simulink model "LKS_tcp11"  (R2024b)
settings: Solver=VariableStepAuto  StartTime=0.0  StopTime=100  RelTol=1e-3
libraries: simulink x3, simulink_extras x3, instrumentlib x1
settings Model: Creator=28509  LastModifiedBy=zc
settings DataIOCC: SaveFormat=Array  ReturnWorkspaceOutputs=off

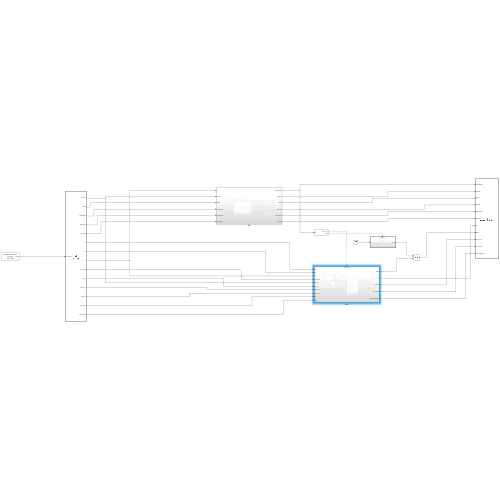
[thumbnail: Simulink's stored preview of the top-level diagram]
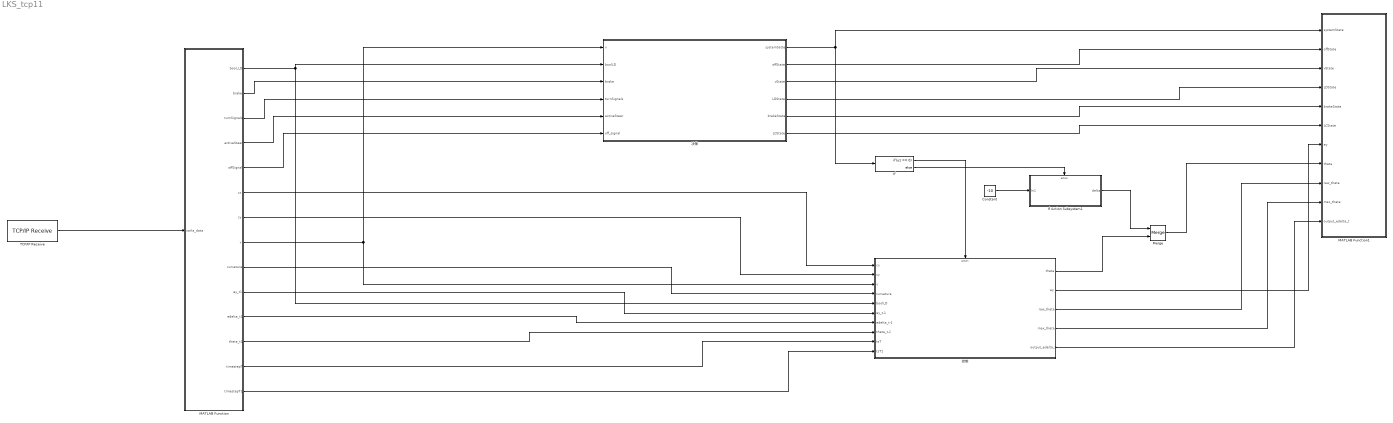
== system LKS_tcp11 ==
  Constant : Constant  Value=-10
  If : If  IfExpression=u1 == 0
  If Action Subsystem1 : Subsystem  TreatAsAtomicUnit=on
  MATLAB Function : MATLAB Function  TreatAsAtomicUnit=on
  MATLAB Function1 : MATLAB Function  TreatAsAtomicUnit=on
  Merge : Merge
  TCP/IP Receive : instrumentlib/TCP//IP Receive  Host=127.0.0.1  Port=25026  DataSize=[ 1, 191]  DataType=double  ASCIIFormatting=%f  Terminator=LF  CustomTerminator=10  ByteOrder=little-endian  EnableBlockingMode=on  Timeout=5  SampleTime=0.01  SimulateUsing=Interpreted execution
  决策 : Subsystem
  控制 : Subsystem  TreatAsAtomicUnit=on
  wires:
  控制/1(theta) -> Merge/2
  MATLAB Function/2(brake) -> 决策/3(brake)
  MATLAB Function/3(turnSignals) -> 决策/4(turnSignals)
  MATLAB Function/4(activeSteer) -> 决策/5(activeSteer)
  决策/1(systemSatte) -> If/1, MATLAB Function1/1(systemState)
  If/1 -> 控制/Action
  MATLAB Function/7(cy) -> 控制/2(cy)
  If/2 -> If Action Subsystem1/Action
  Constant/1 -> If Action Subsystem1/1(In1)
  If Action Subsystem1/1(delta) -> Merge/1
  Merge/1 -> MATLAB Function1/8(theta)
  MATLAB Function/5(offSignal) -> 决策/6(off_signal)
  TCP/IP Receive/1 -> MATLAB Function/1(carla_data)
  MATLAB Function/8(v) -> 决策/1(v), 控制/3(v)
  决策/2(offState) -> MATLAB Function1/2(offState)
  决策/3(vState) -> MATLAB Function1/3(vState)
  决策/4(LDState) -> MATLAB Function1/4(LDState)
  决策/5(brakeState) -> MATLAB Function1/5(brakeState)
  决策/6(LCState) -> MATLAB Function1/6(LCState)
  控制/2(ey) -> MATLAB Function1/7(ey)
  控制/3(raw_theta) -> MATLAB Function1/9(raw_theta)
  控制/4(max_theta) -> MATLAB Function1/10(max_theta)
  MATLAB Function/6(cx) -> 控制/1(cx)
  MATLAB Function/9(curvature) -> 控制/4(curvature)
  MATLAB Function/1(bool_LD) -> 决策/2(boolLD), 控制/5(boolLD)
  控制/5(output_edelta_t) -> MATLAB Function1/11(output_edelta_t)
  MATLAB Function/10(ey_t1) -> 控制/6(ey_t-1)
  MATLAB Function/11(edelta_t1) -> 控制/7(edelta_t-1)
  MATLAB Function/12(theta_t1) -> 控制/8(theta_t-1)
  MATLAB Function/13(timestepT) -> 控制/9(tsT)
  MATLAB Function/14(timestepT1) -> 控制/10(tsT1)

== system LKS_tcp11/If Action Subsystem1 ==
  In1 : Inport
  Action Port : ActionPort  ActionPortLabel=else
  delta : Outport
  wires:
  In1/1 -> delta/1

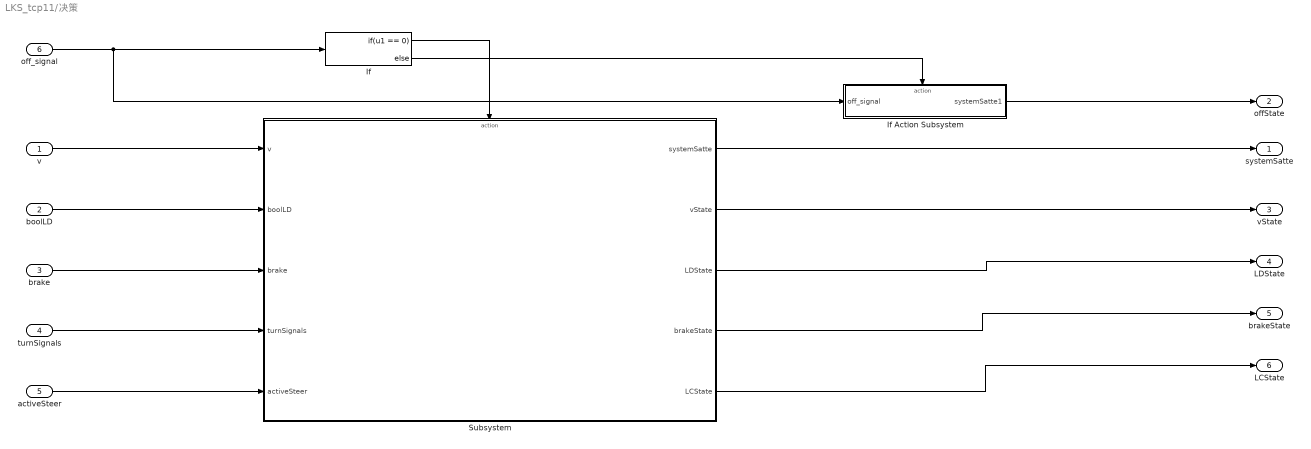
== system LKS_tcp11/决策 ==
  v : Inport
  boolLD : Inport  Port=2
  brake : Inport  Port=3  OutDataTypeStr=double
  turnSignals : Inport  Port=4
  activeSteer : Inport  Port=5
  off_signal : Inport  Port=6
  If : If  IfExpression=u1 == 0
  If Action Subsystem : Subsystem  TreatAsAtomicUnit=on
  Subsystem : Subsystem
  systemSatte : Outport
  offState : Outport  Port=2
  vState : Outport  Port=3
  LDState : Outport  Port=4
  brakeState : Outport  Port=5
  LCState : Outport  Port=6
  wires:
  v/1 -> Subsystem/1(v)
  boolLD/1 -> Subsystem/2(boolLD)
  brake/1 -> Subsystem/3(brake)
  turnSignals/1 -> Subsystem/4(turnSignals)
  activeSteer/1 -> Subsystem/5(activeSteer)
  Subsystem/1(systemSatte) -> systemSatte/1
  If/1 -> Subsystem/Action
  If/2 -> If Action Subsystem/Action
  If Action Subsystem/1(systemSatte1) -> offState/1
  off_signal/1 -> If Action Subsystem/1(off_signal), If/1
  Subsystem/5(LCState) -> LCState/1
  Subsystem/4(brakeState) -> brakeState/1
  Subsystem/2(vState) -> vState/1
  Subsystem/3(LDState) -> LDState/1

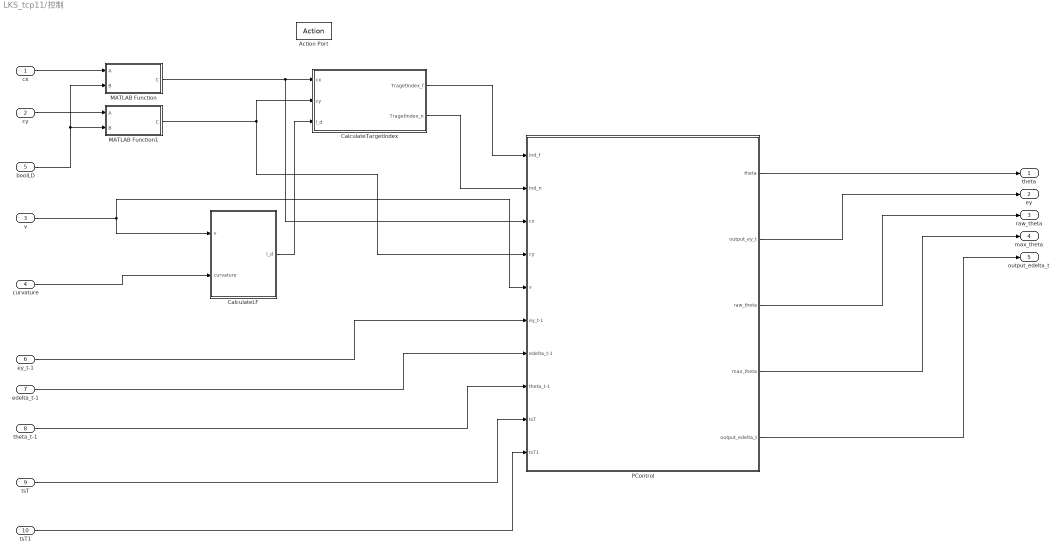
== system LKS_tcp11/控制 ==
  cx : Inport
  cy : Inport  Port=2
  v : Inport  Port=3
  curvature : Inport  Port=4
  boolLD : Inport  Port=5
  ey_t-1 : Inport  Port=6
  edelta_t-1 : Inport  Port=7
  theta_t-1 : Inport  Port=8
  tsT : Inport  Port=9
  tsT1 : Inport  Port=10
  Action Port : ActionPort  ActionPortLabel=if(u1 == 0)
  CalculateLF : Subsystem
  CalculateTargetIndex : Subsystem
  MATLAB Function : MATLAB Function  TreatAsAtomicUnit=on
  MATLAB Function1 : MATLAB Function  TreatAsAtomicUnit=on
  PControl : Subsystem
  theta : Outport  VectorParamsAs1DForOutWhenUnconnected=off
  ey : Outport  Port=2  VectorParamsAs1DForOutWhenUnconnected=off
  raw_theta : Outport  Port=3  VectorParamsAs1DForOutWhenUnconnected=off
  max_theta : Outport  Port=4  VectorParamsAs1DForOutWhenUnconnected=off
  output_edelta_t : Outport  Port=5  VectorParamsAs1DForOutWhenUnconnected=off
  wires:
  PControl/1(theta) -> theta/1
  CalculateLF/1(l_d) -> CalculateTargetIndex/3(l_d)
  CalculateTargetIndex/2(TragetIndex_n) -> PControl/2(ind_n)
  v/1 -> PControl/5(v), CalculateLF/1(v)
  PControl/2(output_ey_t) -> ey/1
  PControl/3(raw_theta) -> raw_theta/1
  PControl/4(max_theta) -> max_theta/1
  curvature/1 -> CalculateLF/2(curvature)
  cx/1 -> MATLAB Function/1(A)
  MATLAB Function/1(C) -> PControl/3(cx), CalculateTargetIndex/1(cx)
  cy/1 -> MATLAB Function1/1(A)
  MATLAB Function1/1(C) -> PControl/4(cy), CalculateTargetIndex/2(cy)
  boolLD/1 -> MATLAB Function/2(B), MATLAB Function1/2(B)
  CalculateTargetIndex/1(TragetIndex_f) -> PControl/1(ind_f)
  ey_t-1/1 -> PControl/6(ey_t-1)
  edelta_t-1/1 -> PControl/7(edelta_t-1)
  theta_t-1/1 -> PControl/8(theta_t-1)
  PControl/5(output_edelta_t) -> output_edelta_t/1
  tsT/1 -> PControl/9(tsT)
  tsT1/1 -> PControl/10(tsT1)

== system LKS_tcp11/决策/If Action Subsystem ==
  off_signal : Inport
  Action Port : ActionPort  ActionPortLabel=else
  systemSatte1 : Outport
  wires:
  off_signal/1 -> systemSatte1/1

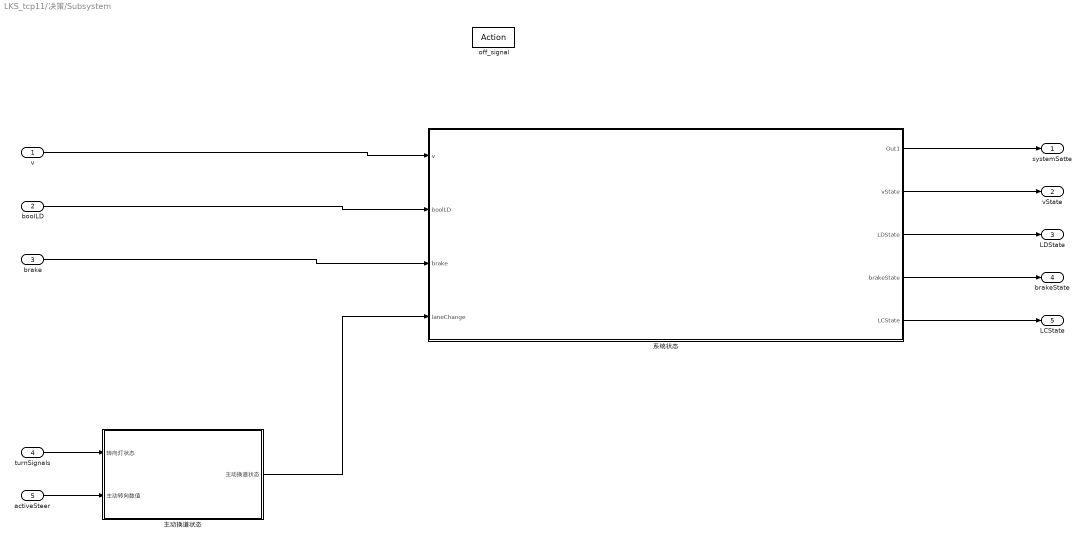
== system LKS_tcp11/决策/Subsystem ==
  v : Inport
  boolLD : Inport  Port=2
  brake : Inport  Port=3  OutDataTypeStr=double
  turnSignals : Inport  Port=4
  activeSteer : Inport  Port=5
  off_signal : ActionPort  ActionPortLabel=if(u1 == 0)
  主动换道状态 : Subsystem
  系统状态 : Subsystem
  systemSatte : Outport
  vState : Outport  Port=2
  LDState : Outport  Port=3
  brakeState : Outport  Port=4
  LCState : Outport  Port=5
  wires:
  v/1 -> 系统状态/1(v)
  主动换道状态/1(主动换道状态) -> 系统状态/4(laneChange)
  turnSignals/1 -> 主动换道状态/1(转向灯状态)
  activeSteer/1 -> 主动换道状态/2(主动转向数值)
  boolLD/1 -> 系统状态/2(boolLD)
  brake/1 -> 系统状态/3(brake)
  系统状态/1(Out1) -> systemSatte/1
  系统状态/2(vState) -> vState/1
  系统状态/3(LDState) -> LDState/1
  系统状态/4(brakeState) -> brakeState/1
  系统状态/5(LCState) -> LCState/1

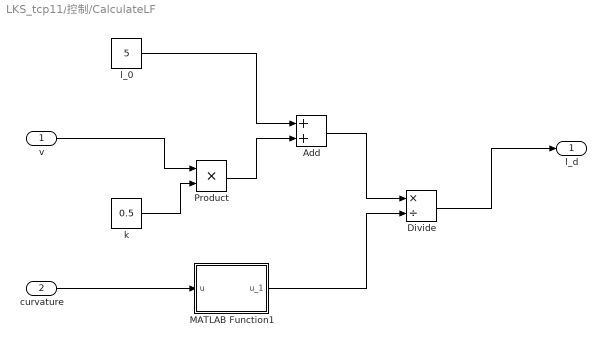
== system LKS_tcp11/控制/CalculateLF ==
  v : Inport
  curvature : Inport  Port=2
  Add : Sum
  Divide : Product  Inputs=*/
  MATLAB Function1 : MATLAB Function  TreatAsAtomicUnit=on
  Product : Product
  k : Constant  Value=0.5
  l_0 : Constant  Value=5
  l_d : Outport
  wires:
  v/1 -> Product/1
  k/1 -> Product/2
  l_0/1 -> Add/1
  Product/1 -> Add/2
  Divide/1 -> l_d/1
  curvature/1 -> MATLAB Function1/1(u)
  Add/1 -> Divide/1
  MATLAB Function1/1(u_1) -> Divide/2

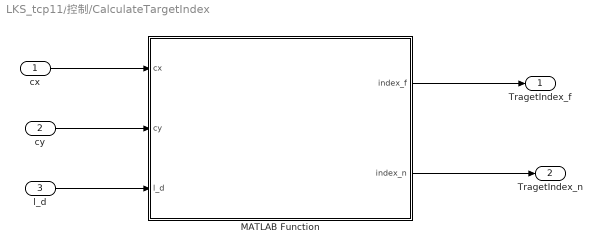
== system LKS_tcp11/控制/CalculateTargetIndex ==
  cx : Inport
  cy : Inport  Port=2
  l_d : Inport  Port=3
  MATLAB Function : MATLAB Function  TreatAsAtomicUnit=on
  TragetIndex_f : Outport
  TragetIndex_n : Outport  Port=2
  wires:
  cx/1 -> MATLAB Function/1(cx)
  cy/1 -> MATLAB Function/2(cy)
  l_d/1 -> MATLAB Function/3(l_d)
  MATLAB Function/2(index_n) -> TragetIndex_n/1
  MATLAB Function/1(index_f) -> TragetIndex_f/1

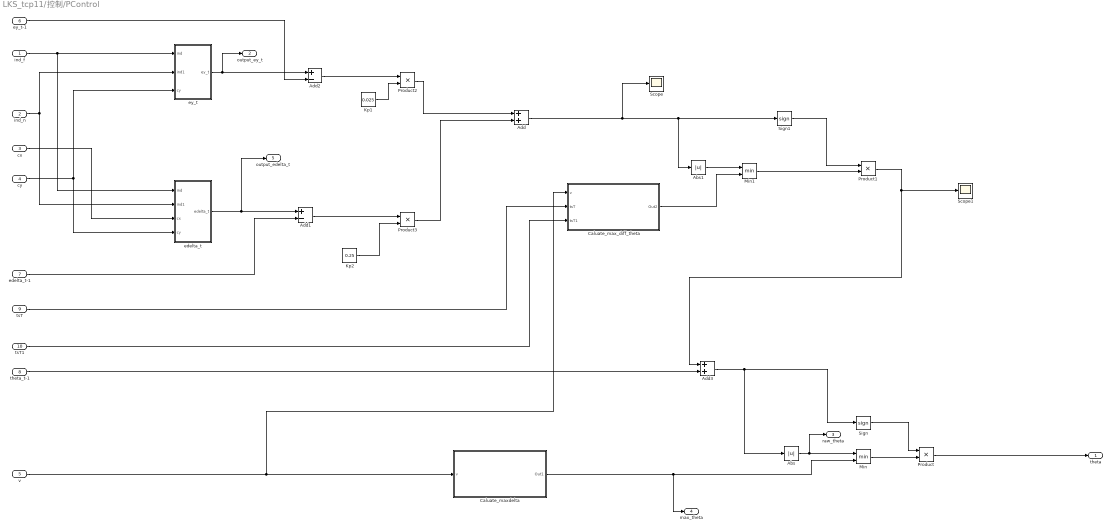
== system LKS_tcp11/控制/PControl ==
  ind_f : Inport
  ind_n : Inport  Port=2
  cx : Inport  Port=3
  cy : Inport  Port=4
  v : Inport  Port=5
  ey_t-1 : Inport  Port=6
  edelta_t-1 : Inport  Port=7
  theta_t-1 : Inport  Port=8
  tsT : Inport  Port=9
  tsT1 : Inport  Port=10
  Abs : Abs  SaturateOnIntegerOverflow=off
  Abs1 : Abs  SaturateOnIntegerOverflow=off
  Add : Sum
  Add1 : Sum  Inputs=+-
  Add2 : Sum  Inputs=+-
  Add3 : Sum
  Caluate_max_diff_theta : Subsystem
  Caluate_maxdelta : Subsystem
  Kp1 : Constant  Value=0.025
  Kp2 : Constant  Value=0.25
  Min : MinMax  Inputs=2
  Min1 : MinMax  Inputs=2
  Product{,1..3} (4 alike) : Product
  Scope : Scope
  Scope1 : Scope
  Sign : Signum
  Sign1 : Signum
  edelta_t : Subsystem
  ey_t : Subsystem
  theta : Outport  VectorParamsAs1DForOutWhenUnconnected=off
  output_ey_t : Outport  Port=2  VectorParamsAs1DForOutWhenUnconnected=off
  raw_theta : Outport  Port=3  VectorParamsAs1DForOutWhenUnconnected=off
  max_theta : Outport  Port=4  VectorParamsAs1DForOutWhenUnconnected=off
  output_edelta_t : Outport  Port=5  VectorParamsAs1DForOutWhenUnconnected=off
  wires:
  Sign/1 -> Product/1
  Min/1 -> Product/2
  Abs/1 -> raw_theta/1, Min/1
  Kp1/1 -> Product2/2
  Product2/1 -> Add/1
  Product3/1 -> Add/2
  Caluate_maxdelta/1(Out1) -> Min/2, max_theta/1
  cy/1 -> edelta_t/4(cy), ey_t/3(cy)
  ind_f/1 -> edelta_t/1(ind), ey_t/1(ind)
  ind_n/1 -> edelta_t/2(ind1), ey_t/2(ind1)
  Kp2/1 -> Product3/2
  cx/1 -> edelta_t/3(cx)
  edelta_t/1(edelta_t) -> output_edelta_t/1, Add1/1
  ey_t/1(ey_t) -> Add2/1, output_ey_t/1
  ey_t-1/1 -> Add2/2
  edelta_t-1/1 -> Add1/2
  Add2/1 -> Product2/1
  Add1/1 -> Product3/1
  Add3/1 -> Abs/1, Sign/1
  Product/1 -> theta/1
  theta_t-1/1 -> Add3/2
  Sign1/1 -> Product1/1
  Min1/1 -> Product1/2
  Abs1/1 -> Min1/1
  Caluate_max_diff_theta/1(Out2) -> Min1/2
  v/1 -> Caluate_maxdelta/1(v), Caluate_max_diff_theta/1(v)
  tsT/1 -> Caluate_max_diff_theta/2(tsT)
  tsT1/1 -> Caluate_max_diff_theta/3(tsT1)
  Add/1 -> Scope/1, Sign1/1, Abs1/1
  Product1/1 -> Scope1/1, Add3/1

== system LKS_tcp11/决策/Subsystem/主动换道状态 ==
  转向灯状态 : Inport
  主动转向数值 : Inport  Port=2
  Abs : Abs  SaturateOnIntegerOverflow=off
  Add : Sum
  Compare To Constant : simulink/Logic and Bit Operations/Compare To Constant  relop=>=  const=0.05  OutDataTypeStr=boolean
  主动换道状态 : Outport
  wires:
  Compare To Constant/1 -> Add/2
  Add/1 -> 主动换道状态/1
  转向灯状态/1 -> Add/1
  主动转向数值/1 -> Abs/1
  Abs/1 -> Compare To Constant/1

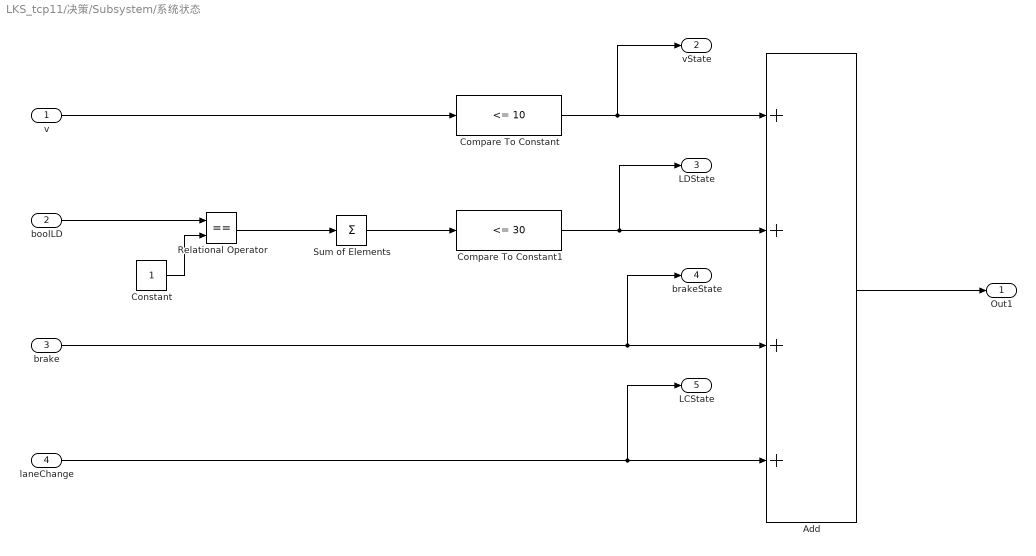
== system LKS_tcp11/决策/Subsystem/系统状态 ==
  v : Inport
  boolLD : Inport  Port=2
  brake : Inport  Port=3
  laneChange : Inport  Port=4
  Add : Sum  Inputs=++++
  Compare To Constant : simulink/Logic and Bit Operations/Compare To Constant  relop=<=  const=10  OutDataTypeStr=boolean
  Compare To Constant1 : simulink/Logic and Bit Operations/Compare To Constant  relop=<=  const=30  OutDataTypeStr=boolean
  Constant : Constant
  Relational Operator : RelationalOperator  Operator===  OutDataTypeStr=boolean  RndMeth=Simplest  InputSameDT=off
  Sum of Elements : Sum  Inputs=+
  Out1 : Outport
  vState : Outport  Port=2
  LDState : Outport  Port=3
  brakeState : Outport  Port=4
  LCState : Outport  Port=5
  wires:
  boolLD/1 -> Relational Operator/1
  Constant/1 -> Relational Operator/2
  Relational Operator/1 -> Sum of Elements/1
  Add/1 -> Out1/1
  Compare To Constant/1 -> vState/1, Add/1
  Compare To Constant1/1 -> LDState/1, Add/2
  brake/1 -> brakeState/1, Add/3
  laneChange/1 -> LCState/1, Add/4
  v/1 -> Compare To Constant/1
  Sum of Elements/1 -> Compare To Constant1/1

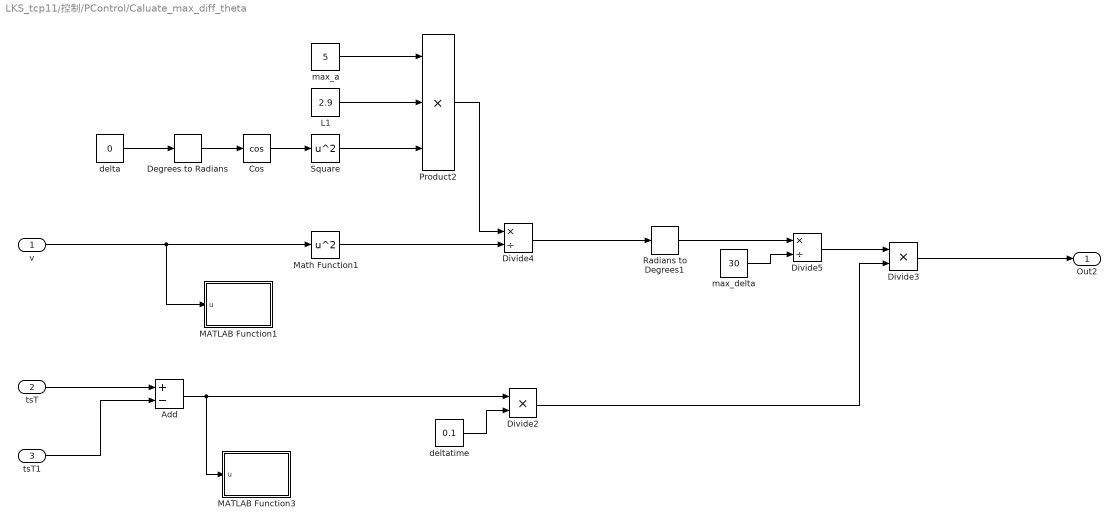
== system LKS_tcp11/控制/PControl/Caluate_max_diff_theta ==
  v : Inport
  tsT : Inport  Port=2
  tsT1 : Inport  Port=3
  Add : Sum  Inputs=+-
  Cos : Trigonometry  Operator=cos
  Degrees to Radians : simulink_extras/Transformations/Degrees to Radians
  Divide2 : Product  Inputs=**
  Divide3 : Product  Inputs=**
  Divide4 : Product  Inputs=*/
  Divide5 : Product  Inputs=*/
  L1 : Constant  Value=2.9
  MATLAB Function1 : MATLAB Function  TreatAsAtomicUnit=on
  MATLAB Function3 : MATLAB Function  TreatAsAtomicUnit=on
  Math Function1 : Math  Operator=square
  Product2 : Product  Inputs=3
  Radians to Degrees1 : simulink_extras/Transformations/Radians to Degrees
  Square : Math  Operator=square
  delta : Constant  Value=0
  deltatime : Constant  Value=0.1
  max_a : Constant  Value=5
  max_delta : Constant  Value=30
  Out2 : Outport
  wires:
  tsT/1 -> Add/1
  tsT1/1 -> Add/2
  Add/1 -> MATLAB Function3/1(u), Divide2/1
  deltatime/1 -> Divide2/2
  max_a/1 -> Product2/1
  Math Function1/1 -> Divide4/2
  Square/1 -> Product2/3
  Divide3/1 -> Out2/1
  Divide4/1 -> Radians to Degrees1/1
  L1/1 -> Product2/2
  max_delta/1 -> Divide5/2
  Radians to Degrees1/1 -> Divide5/1
  Cos/1 -> Square/1
  Degrees to Radians/1 -> Cos/1
  Product2/1 -> Divide4/1
  Divide2/1 -> Divide3/2
  Divide5/1 -> Divide3/1
  v/1 -> MATLAB Function1/1(u), Math Function1/1
  delta/1 -> Degrees to Radians/1

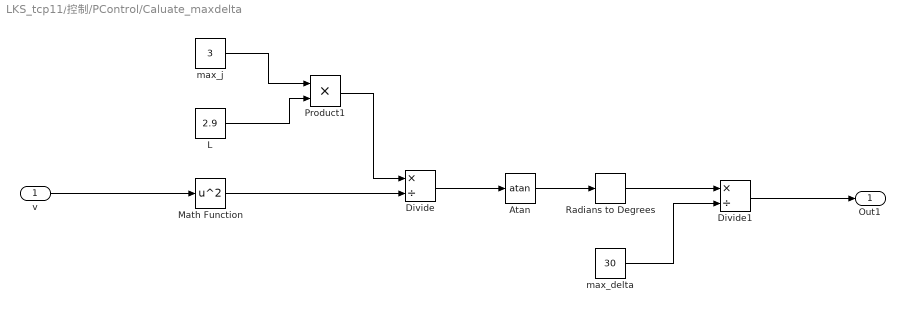
== system LKS_tcp11/控制/PControl/Caluate_maxdelta ==
  v : Inport
  Atan : Trigonometry  Operator=atan
  Divide : Product  Inputs=*/
  Divide1 : Product  Inputs=*/
  L : Constant  Value=2.9
  Math Function : Math  Operator=square
  Product1 : Product
  Radians to Degrees : simulink_extras/Transformations/Radians to Degrees
  max_delta : Constant  Value=30
  max_j : Constant  Value=3
  Out1 : Outport
  wires:
  L/1 -> Product1/2
  v/1 -> Math Function/1
  Divide/1 -> Atan/1
  max_j/1 -> Product1/1
  Divide1/1 -> Out1/1
  Product1/1 -> Divide/1
  max_delta/1 -> Divide1/2
  Math Function/1 -> Divide/2
  Radians to Degrees/1 -> Divide1/1
  Atan/1 -> Radians to Degrees/1

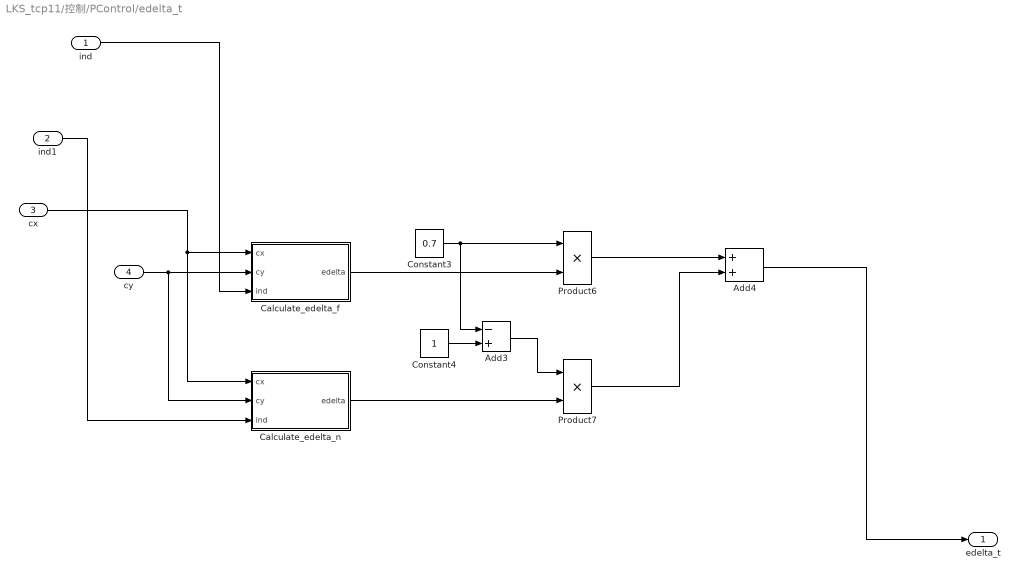
== system LKS_tcp11/控制/PControl/edelta_t ==
  ind : Inport
  ind1 : Inport  Port=2
  cx : Inport  Port=3
  cy : Inport  Port=4
  Add3 : Sum  Inputs=-+
  Add4 : Sum
  Calculate_edelta_f : Subsystem
  Calculate_edelta_n : Subsystem
  Constant3 : Constant  Value=0.7
  Constant4 : Constant
  Product6 : Product
  Product7 : Product
  edelta_t : Outport
  wires:
  Product6/1 -> Add4/1
  Constant4/1 -> Add3/2
  Constant3/1 -> Add3/1, Product6/1
  Add3/1 -> Product7/1
  Calculate_edelta_n/1(edelta) -> Product7/2
  ind/1 -> Calculate_edelta_f/3(ind)
  Product7/1 -> Add4/2
  ind1/1 -> Calculate_edelta_n/3(ind)
  Calculate_edelta_f/1(edelta) -> Product6/2
  cy/1 -> Calculate_edelta_n/2(cy), Calculate_edelta_f/2(cy)
  Add4/1 -> edelta_t/1
  cx/1 -> Calculate_edelta_n/1(cx), Calculate_edelta_f/1(cx)

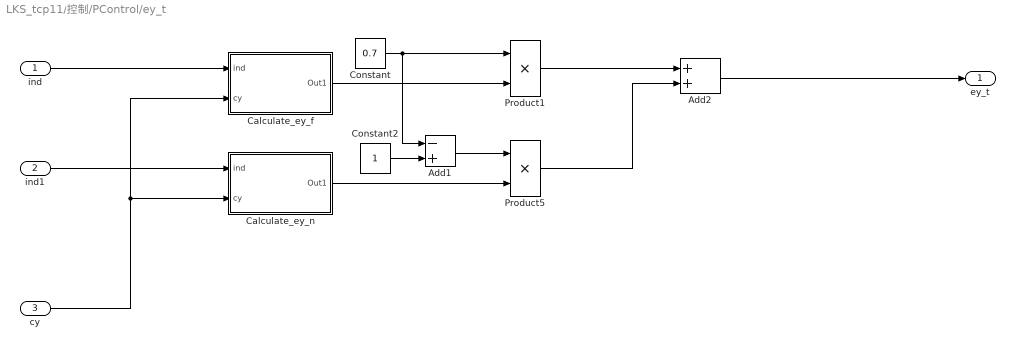
== system LKS_tcp11/控制/PControl/ey_t ==
  ind : Inport
  ind1 : Inport  Port=2
  cy : Inport  Port=3
  Add1 : Sum  Inputs=-+
  Add2 : Sum
  Calculate_ey_f : Subsystem
  Calculate_ey_n : Subsystem
  Constant : Constant  Value=0.7
  Constant2 : Constant
  Product1 : Product
  Product5 : Product
  ey_t : Outport
  wires:
  Constant2/1 -> Add1/2
  ind1/1 -> Calculate_ey_n/1(ind)
  Product1/1 -> Add2/1
  Product5/1 -> Add2/2
  Constant/1 -> Add1/1, Product1/1
  Add1/1 -> Product5/1
  Calculate_ey_f/1(Out1) -> Product1/2
  Calculate_ey_n/1(Out1) -> Product5/2
  cy/1 -> Calculate_ey_n/2(cy), Calculate_ey_f/2(cy)
  Add2/1 -> ey_t/1
  ind/1 -> Calculate_ey_f/1(ind)

== system LKS_tcp11/控制/PControl/edelta_t/Calculate_edelta_f ==
  cx : Inport
  cy : Inport  Port=2
  ind : Inport  Port=3
  Constant : Constant  Value=2
  MATLAB Function : MATLAB Function  TreatAsAtomicUnit=on
  edelta : Outport
  wires:
  ind/1 -> MATLAB Function/3(i)
  cy/1 -> MATLAB Function/2(y)
  MATLAB Function/1(edelta) -> edelta/1
  cx/1 -> MATLAB Function/1(x)
  Constant/1 -> MATLAB Function/4(k)

== system LKS_tcp11/控制/PControl/edelta_t/Calculate_edelta_n ==
  cx : Inport
  cy : Inport  Port=2
  ind : Inport  Port=3
  Constant : Constant  Value=2
  MATLAB Function : MATLAB Function  TreatAsAtomicUnit=on
  edelta : Outport
  wires:
  ind/1 -> MATLAB Function/3(i)
  cy/1 -> MATLAB Function/2(y)
  MATLAB Function/1(edelta) -> edelta/1
  cx/1 -> MATLAB Function/1(x)
  Constant/1 -> MATLAB Function/4(k)

== system LKS_tcp11/控制/PControl/ey_t/Calculate_ey_f ==
  ind : Inport
  cy : Inport  Port=2
  Index Vector2 : MultiPortSwitch  Inputs=1  SaturateOnIntegerOverflow=off  InputSameDT=off
  Out1 : Outport
  wires:
  ind/1 -> Index Vector2/1
  cy/1 -> Index Vector2/2
  Index Vector2/1 -> Out1/1

== system LKS_tcp11/控制/PControl/ey_t/Calculate_ey_n ==
  ind : Inport
  cy : Inport  Port=2
  Index Vector2 : MultiPortSwitch  Inputs=1  SaturateOnIntegerOverflow=off  InputSameDT=off
  Out1 : Outport
  wires:
  ind/1 -> Index Vector2/1
  cy/1 -> Index Vector2/2
  Index Vector2/1 -> Out1/1

== matlab function LKS_tcp11/控制/MATLAB Function1 ==
  data: A input; C output; B input
function C = filterArray(A, B)
% 输入A和B都是固定大小1x60，输出C最大为1x60，但实际长度取决于B中1的个数
% 将B转换为逻辑索引
mask = logical(B);
% 提取对应元素
temp = A(mask);   % temp是可变长度的向量

% 初始化输出为最大可能长度的向量（用零填充，但实际只使用前一部分）
maxLen = length(A);
C = zeros(1, maxLen);
len = length(temp);
if len > 0
    C(1:len) = temp;
end
end

== matlab function LKS_tcp11/控制/PControl/Caluate_max_diff_theta/MATLAB Function3 ==
  data: u input
function fcn(u)
disp("diff_ts")
disp(u)

== matlab function LKS_tcp11/控制/PControl/Caluate_max_diff_theta/MATLAB Function1 ==
  data: u input
function fcn(u)
disp("vvvvvv")
disp(u)

== matlab function LKS_tcp11/控制/CalculateTargetIndex/MATLAB Function ==
  data: index_f output; index_n output; cx input; cy input; l_d input
function [index_f, index_n]  = calc_target_index(cx, cy, l_d)
    N =  length(cx);
    for j = 1:N
        index_n = j;
        if cx(j)>0
            break;
        end
    end

    for i = 1:N
        delta_l =  sqrt((cx(i))^2 + (cy(i))^2);
        index_f = i;
        if delta_l >= l_d
            break;
        end
    end
end

== matlab function LKS_tcp11/控制/PControl/edelta_t/Calculate_edelta_f/MATLAB Function ==
  data: x input; y input; edelta output; i input; k input
function edelta = calculate_heading_linear_fit(x, y, i, k)
    % 滑动窗口线性拟合计算航向角（适配x/y独立向量输入）
    % 输入参数：
    %   x         - 路点x坐标向量（行/列向量均可），长度为N
    %   y         - 路点y坐标向量（行/列向量均可），长度需与x一致
    %   i         - 当前路点的索引（MATLAB索引从1开始）
    %   k         - 窗口半宽（可选，默认值2，即使用5个点拟合）
    % 输出参数：
    %   theta     - 航向角（弧度），范围[-π, π]
    

    N = length(x);  % 路点总数
    
    % ========== 设置默认参数 ==========
    if nargin < 4  % 未传入k时，默认窗口半宽为2
        k = 2;
    end
    
    % ========== 处理窗口边界（避免越界） ==========
    left = max(1, i - k);    % 左边界不小于1
    right = min(N, i + k);   % 右边界不大于路点总数
    
    % ========== 提取窗口内的x/y子向量（统一转为列向量方便计算） ==========
    x_window = x(left:right);
    y_window = y(left:right);
    x_window = x_window(:);  % 转为列向量
    y_window = y_window(:);  % 转为列向量
    
    % ========== 最小二乘拟合直线 y = a*x + b ==========
    % 构造设计矩阵 X = [x, 1]（列向量形式）
    X = [x_window, ones(length(x_window), 1)];
    % MATLAB反斜杠运算符求解最小二乘（高效且稳定）
    coeffs = X \ y_window;
    a = coeffs(1);  % 拟合直线的斜率
    % b = coeffs(2); % 截距，航向角计算无需用到
    
    % ========== 计算航向角 ==========
    % 直线方向向量为(1, a)，用atan2(dy, dx)计算角度（范围[-π, π]）
    dx = 1.0;
    dy = a;
    edelta = atan2(dy, dx);
end

== matlab function LKS_tcp11/MATLAB Function1 ==
  data: systemState input; offState input; vState input; LDState input; brakeState input; LCState input; ey input; theta input; raw_theta input; max_theta input; output_edelta_t input
function send_simulink_data(systemState, offState,vState,LDState,brakeState,LCState,ey,theta,raw_theta,max_theta,output_edelta_t)

        host = '127.0.0.1';
        port = 25028;
    
        persistent tcpClient
        if isempty(tcpClient)
            tcpClient = tcpclient(host, port, 'Timeout', 5);
        end
    
    
        data = typecast([double(systemState),double(offState),double(vState),double(LDState),double(brakeState),double(LCState),double(ey),double(theta),double(raw_theta),double(max_theta),double(output_edelta_t)], 'uint8');
        % Write the byte data to the TCP stream
        write(tcpClient, data);
        %disp("send data successfully data len");
end

== matlab function LKS_tcp11/控制/PControl/edelta_t/Calculate_edelta_n/MATLAB Function ==
  data: x input; y input; edelta output; i input; k input
function edelta = calculate_heading_linear_fit(x, y, i, k)
    % 滑动窗口线性拟合计算航向角（适配x/y独立向量输入）
    % 输入参数：
    %   x         - 路点x坐标向量（行/列向量均可），长度为N
    %   y         - 路点y坐标向量（行/列向量均可），长度需与x一致
    %   i         - 当前路点的索引（MATLAB索引从1开始）
    %   k         - 窗口半宽（可选，默认值2，即使用5个点拟合）
    % 输出参数：
    %   theta     - 航向角（弧度），范围[-π, π]
    
    % ========== 输入合法性检查 ==========

    N = length(x);  % 路点总数

    
    % ========== 设置默认参数 ==========
    if nargin < 4  % 未传入k时，默认窗口半宽为2
        k = 2;
    end
    
    % ========== 处理窗口边界（避免越界） ==========
    left = max(1, i - k);    % 左边界不小于1
    right = min(N, i + k);   % 右边界不大于路点总数
    
    % ========== 提取窗口内的x/y子向量（统一转为列向量方便计算） ==========
    x_window = x(left:right);
    y_window = y(left:right);
    x_window = x_window(:);  % 转为列向量
    y_window = y_window(:);  % 转为列向量
    
    % ========== 最小二乘拟合直线 y = a*x + b ==========
    % 构造设计矩阵 X = [x, 1]（列向量形式）
    X = [x_window, ones(length(x_window), 1)];
    % MATLAB反斜杠运算符求解最小二乘（高效且稳定）
    coeffs = X \ y_window;
    a = coeffs(1);  % 拟合直线的斜率
    % b = coeffs(2); % 截距，航向角计算无需用到
    
    % ========== 计算航向角 ==========
    % 直线方向向量为(1, a)，用atan2(dy, dx)计算角度（范围[-π, π]）
    dx = 1.0;
    dy = a;
    edelta = atan2(dy, dx);
end

== matlab function LKS_tcp11/MATLAB Function ==
  data: bool_LD output; brake output; turnSignals output; activeSteer output; offSignal output; carla_data input; cx output; cy output; v output; curvature output; ey_t1 output; edelta_t1 output; theta_t1 output; timestepT output; timestepT1 output
function [bool_LD,brake,turnSignals,activeSteer,offSignal,cx,cy,v,curvature,ey_t1,edelta_t1,theta_t1,timestepT,timestepT1] = tcp2input(carla_data)
    %disp("carla_data");
    %disp(length(carla_data));
    bool_LD = carla_data(1:60);
    brake = carla_data(61);
    turnSignals = carla_data(62);
    activeSteer = carla_data(63);
    offSignal = carla_data(64);
    %x = carla_data(65);
    %y = carla_data(66);
    v = carla_data(65);
    %disp(v);
    cx = carla_data(66:125);
    cy = carla_data(126:185);
    curvature = carla_data(186);

    ey_t1=carla_data(187);
    edelta_t1=carla_data(188);
    theta_t1=carla_data(189);

    timestepT=carla_data(190);
    timestepT1=carla_data(191);
    
end

== matlab function LKS_tcp11/控制/CalculateLF/MATLAB Function1 ==
  data: u input; u_1 output
function u_1 = fcn(u)
u_1 = 1;
if u == 1
    u_1 = 1.5;
end

== matlab function LKS_tcp11/控制/MATLAB Function ==
  data: A input; C output; B input
function C = filterArray(A, B)
% 输入A和B都是固定大小1x60，输出C最大为1x60，但实际长度取决于B中1的个数
% 将B转换为逻辑索引
mask = logical(B);
% 提取对应元素
temp = A(mask);   % temp是可变长度的向量

% 初始化输出为最大可能长度的向量（用零填充，但实际只使用前一部分）
maxLen = length(A);
C = zeros(1, maxLen);
len = length(temp);
if len > 0
    C(1:len) = temp;
end
end
